simulink subsystem "biasEstimation"  (R2026a)
settings: Solver=VariableStepAuto
undefined symbols (not defined in the file or in its folder): flightMode
libraries: simulink x1
settings Model: Creator=maxhu  LastModifiedBy=maxhu

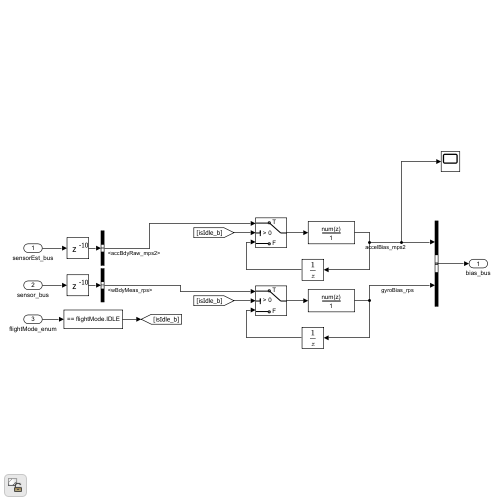
[thumbnail: Simulink's stored preview of the top-level diagram]
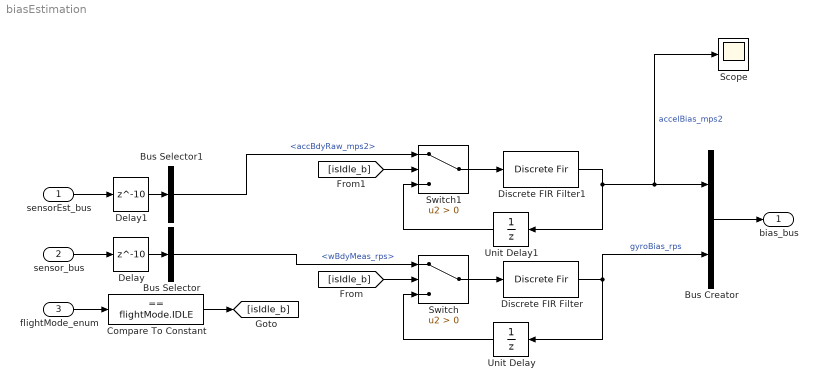
== system biasEstimation ==
  sensorEst_bus : Inport
  sensor_bus : Inport  Port=2
  flightMode_enum : Inport  Port=3
  Bus Creator : BusCreator  Inputs=2
  Bus Selector : BusSelector  OutputSignals=wBdyMeas_rps
  Bus Selector1 : BusSelector  OutputSignals=accBdyRaw_mps2
  Compare To Constant : simulink/Logic and Bit Operations/Compare To Constant  relop===  const=flightMode.IDLE  OutDataTypeStr=boolean
  Delay : Delay  DelayLength=10
  Delay1 : Delay  DelayLength=10
  Discrete FIR Filter : DiscreteFir  Coefficients=ones(1,100)/100
  Discrete FIR Filter1 : DiscreteFir  Coefficients=ones(1,100)/100
  Scope : Scope
      settings: ActiveDisplayYMinimum=-0.72246730490352129  ActiveDisplayYMaximum=0.71340977374152392
  Switch : Switch  Criteria=u2 > Threshold  SaturateOnIntegerOverflow=off  InputSameDT=off
  Switch1 : Switch  Criteria=u2 > Threshold  SaturateOnIntegerOverflow=off  InputSameDT=off
  Unit Delay : UnitDelay  SampleTime=-1
  Unit Delay1 : UnitDelay  SampleTime=-1
  bias_bus : Outport
  wires:
  Discrete FIR Filter/1 -> Bus Creator/2, Unit Delay/1  "gyroBias_rps"
  Unit Delay/1 -> Switch/3
  Switch/1 -> Discrete FIR Filter/1
  flightMode_enum/1 -> Compare To Constant/1
  sensor_bus/1 -> Delay/1
  Bus Selector/1 -> Switch/1  "<wBdyMeas_rps>"
  Compare To Constant/1 -> [isIdle_b]
  [isIdle_b] -> Switch/2
  Delay/1 -> Bus Selector/1
  Unit Delay1/1 -> Switch1/3
  Switch1/1 -> Discrete FIR Filter1/1
  [isIdle_b] -> Switch1/2
  Discrete FIR Filter1/1 -> Bus Creator/1, Scope/1, Unit Delay1/1  "accelBias_mps2"
  Bus Creator/1 -> bias_bus/1
  Delay1/1 -> Bus Selector1/1
  Bus Selector1/1 -> Switch1/1  "<accBdyRaw_mps2>"
  sensorEst_bus/1 -> Delay1/1
